simulink model "fixpt_multi_input"  (R2015b)
settings: Solver=FixedStepDiscrete  StartTime=0.0  StopTime=0  FixedStep=1  RelTol=1e-3
settings Model: Creator=y_yama  LastModifiedBy=amatsumo
settings DataIOCC: SaveFormat=Array  SignalLoggingSaveFormat=ModelDataLogs  SaveOutput=off  SignalLogging=off  SaveTime=off
settings OptimizationCC: BlockReduction=off  ConditionallyExecuteInputs=off  DefaultParameterBehavior=Inlined  InlineInvariantSignals=on  ExpressionDepthLimit=2147483647  ZeroExternalMemoryAtStartup=off  ZeroInternalMemoryAtStartup=off  InitFltsAndDblsToZero=on  NoFixptDivByZeroProtection=on  EfficientFloat2IntCast=on  OptimizeModelRefInitCode=on  LifeSpan=1
settings DebuggingCC: UnderspecifiedInitializationDetection=Classic  MergeDetectMultiDrivingBlocksExec=none  SolverPrmCheckMsg=warning  InheritedTsInSrcMsg=none  FcnCallInpInsideContextMsg=UseLocalSettings  StateNameClashWarn=warning
settings HardwareCC: ProdBitPerPointer=32  ProdLargestAtomicFloat=None  ProdIntDivRoundTo=Undefined  ProdEndianess=Unspecified  ProdWordSize=32  ProdHWDeviceType=ASIC/FPGA->ASIC/FPGA  TargetBitPerPointer=64  TargetLongLongMode=on  TargetIntDivRoundTo=Zero  TargetEndianess=LittleEndian  TargetWordSize=64  TargetHWDeviceType=MATLAB Host  ProdEqTarget=off
settings RTWCC: SystemTargetFile=ert.tlc  GenCodeOnly=on  TemplateMakefile=ert_default_tmf  Description=Real-Time Workshop Embedded Coder (no auto configuration)  GenerateReport=on  IncludeHyperlinkInReport=on  LaunchReport=on
settings CodeAppCC: GenerateComments=off  IgnoreCustomStorageClasses=off  CustomSymbolStrGlobalVar=$N$M  CustomSymbolStrType=$N$R$M  SimulinkBlockComments=off  InternalIdentifier=Classic
settings ERTTargetCC: GenerateSampleERTMain=on  IncludeMdlTerminateFcn=off  SuppressErrorStatus=on  SupportAbsoluteTime=off  SupportNonFinite=off  SupportComplex=off  PurelyIntegerCode=on  InlinedParameterPlacement=NonHierarchical  ERTCustomFileTemplate=example_file_process.tlc
settings ConfigComp: CovModelRefEnable=Off  CovSFcnEnable=off

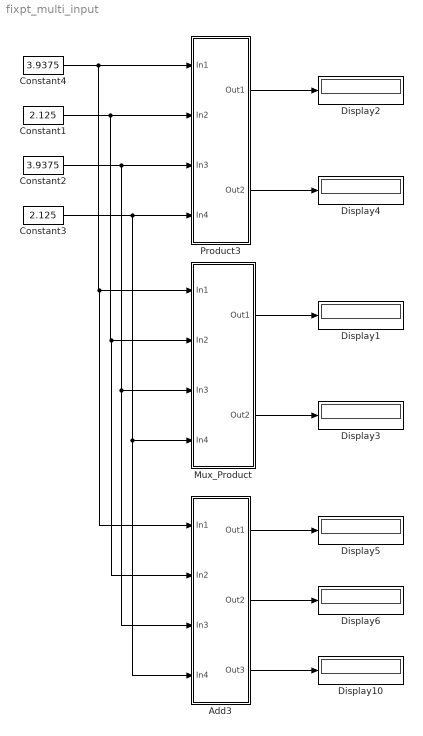
== system fixpt_multi_input ==
  Add3 : Subsystem
  Constant1 : Constant  Value=2.125  OutDataTypeStr=fixdt(1,8,4)  SampleTime=-1
      settings: AttributesFormatString=DataType = %<OutDataTypeStr>
  Constant2 : Constant  Value=3.9375  OutDataTypeStr=fixdt(1,8,4)  SampleTime=-1
      settings: AttributesFormatString=DataType = %<OutDataTypeStr>
  Constant3 : Constant  Value=2.125  OutDataTypeStr=fixdt(1,8,4)  SampleTime=-1
      settings: AttributesFormatString=DataType = %<OutDataTypeStr>
  Constant4 : Constant  Value=3.9375  OutDataTypeStr=fixdt(1,8,4)  SampleTime=-1
      settings: AttributesFormatString=DataType = %<OutDataTypeStr>
  Display{1..6,10} (7 alike) : Display
      settings: AttributesFormatString=Format = %<Format>
  Mux_Product : Subsystem
  Product3 : Subsystem
  wires:
  Constant4/1 -> Product3/1(In1), Add3/1(In1), Mux_Product/1(In1)
  Constant2/1 -> Product3/3(In3), Add3/3(In3), Mux_Product/3(In3)
  Constant3/1 -> Product3/4(In4), Add3/4(In4), Mux_Product/4(In4)
  Mux_Product/1(Out1) -> Display1/1
  Mux_Product/2(Out2) -> Display3/1
  Product3/2(Out2) -> Display4/1
  Product3/1(Out1) -> Display2/1
  Constant1/1 -> Product3/2(In2), Add3/2(In2), Mux_Product/2(In2)
  Add3/1(Out1) -> Display5/1
  Add3/2(Out2) -> Display6/1
  Add3/3(Out3) -> Display10/1

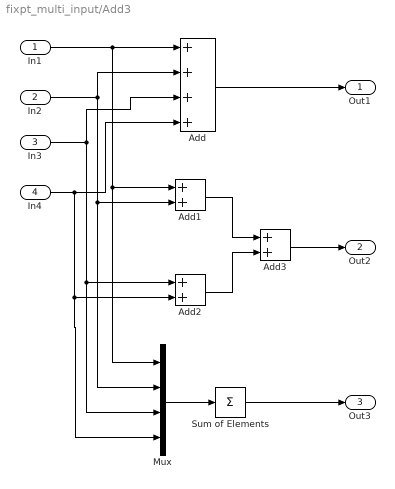
== system fixpt_multi_input/Add3 ==
  In1 : Inport
  In2 : Inport  Port=2
  In3 : Inport  Port=3
  In4 : Inport  Port=4
  Add : Sum  Inputs=++++
      settings: AttributesFormatString=%<AccumDataTypeStr>\n%<OutDataTypeStr>
  Add1 : Sum
      settings: AttributesFormatString=%<AccumDataTypeStr>\n%<OutDataTypeStr>
  Add2 : Sum
      settings: AttributesFormatString=%<AccumDataTypeStr>\n%<OutDataTypeStr>
  Add3 : Sum
      settings: AttributesFormatString=%<AccumDataTypeStr>\n%<OutDataTypeStr>
  Mux : Mux
  Sum of Elements : Sum  Inputs=+
      settings: AttributesFormatString=%<AccumDataTypeStr>\n%<OutDataTypeStr>
  Out1 : Outport
  Out2 : Outport  Port=2
  Out3 : Outport  Port=3
  wires:
  Add/1 -> Out1/1
  In1/1 -> Mux/1, Add1/1, Add/1
  In2/1 -> Mux/2, Add1/2, Add/2
  In4/1 -> Mux/4, Add2/2, Add/4
  In3/1 -> Mux/3, Add2/1, Add/3
  Add1/1 -> Add3/1
  Add2/1 -> Add3/2
  Add3/1 -> Out2/1
  Mux/1 -> Sum of Elements/1
  Sum of Elements/1 -> Out3/1

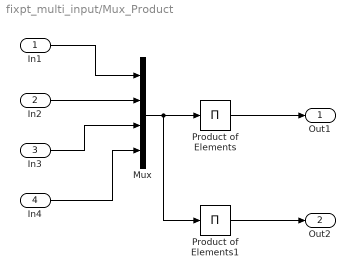
== system fixpt_multi_input/Mux_Product ==
  In1 : Inport
  In2 : Inport  Port=2
  In3 : Inport  Port=3
  In4 : Inport  Port=4
  Mux : Mux
  Product of Elements : Product  Inputs=*  RndMeth=Nearest
      settings: AttributesFormatString=%<OutDataTypeStr>
  Product of Elements1 : Product  Inputs=*  OutDataTypeStr=fixdt(1,32,16)  RndMeth=Nearest
      settings: AttributesFormatString=%<OutDataTypeStr>
  Out1 : Outport
  Out2 : Outport  Port=2
  wires:
  In1/1 -> Mux/1
  Product of Elements/1 -> Out1/1
  Mux/1 -> Product of Elements1/1, Product of Elements/1
  In4/1 -> Mux/4
  In2/1 -> Mux/2
  In3/1 -> Mux/3
  Product of Elements1/1 -> Out2/1

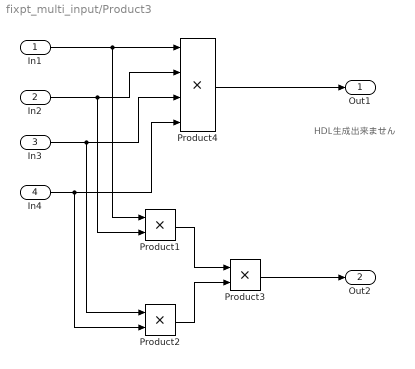
== system fixpt_multi_input/Product3 ==
  note: HDL生成出来ません
  In1 : Inport
  In2 : Inport  Port=2
  In3 : Inport  Port=3
  In4 : Inport  Port=4
  Product1 : Product  RndMeth=Nearest
      settings: AttributesFormatString=%<OutDataTypeStr>
  Product2 : Product  RndMeth=Nearest
      settings: AttributesFormatString=%<OutDataTypeStr>
  Product3 : Product  RndMeth=Nearest
      settings: AttributesFormatString=%<OutDataTypeStr>
  Product4 : Product  Inputs=4  RndMeth=Nearest
      settings: AttributesFormatString=%<OutDataTypeStr>
  Out1 : Outport
  Out2 : Outport  Port=2
  wires:
  Product3/1 -> Out2/1
  Product2/1 -> Product3/2
  Product1/1 -> Product3/1
  In3/1 -> Product2/1, Product4/3
  In4/1 -> Product2/2, Product4/4
  In2/1 -> Product1/2, Product4/2
  In1/1 -> Product4/1, Product1/1
  Product4/1 -> Out1/1
